simulink model "RL_AGENT_SAFE_POLICY"  (R2022b)
settings: Solver=FixedStepAuto  StartTime=0.0  StopTime=10.0  RelTol=1e-3
libraries: rllib x1
settings Model: Creator=Daniel  LastModifiedBy=Daniel
settings SFSimCC: SimTargetLang=C++

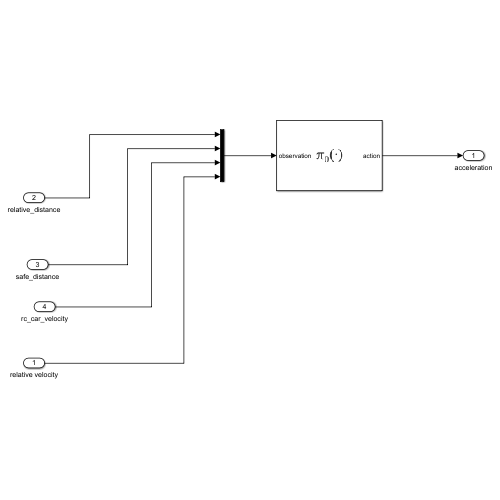
[thumbnail: Simulink's stored preview of the top-level diagram]
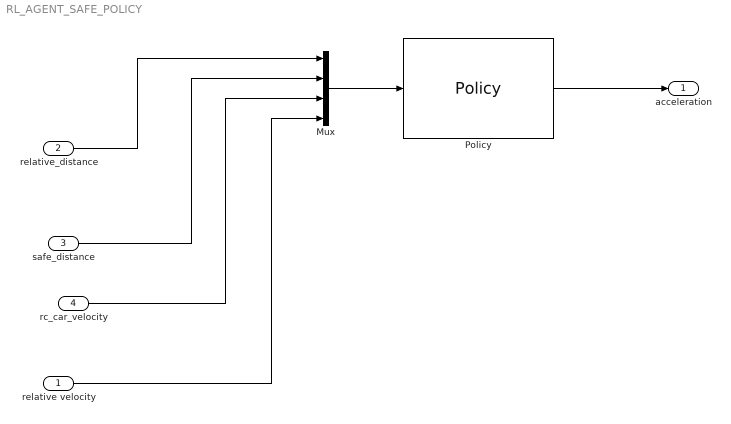
== system RL_AGENT_SAFE_POLICY ==
  relative velocity : Inport
  relative_distance : Inport  Port=2
  safe_distance : Inport  Port=3
  rc_car_velocity : Inport  Port=4
  Mux : Mux
  Policy : rllib/Policy  MATFile=blockAgentData5.mat  SimUsingCodegen=off
  acceleration : Outport
  wires:
  safe_distance/1 -> Mux/2
  relative_distance/1 -> Mux/1
  rc_car_velocity/1 -> Mux/3
  Mux/1 -> Policy/1
  relative velocity/1 -> Mux/4
  Policy/1 -> acceleration/1
